simulink model "pitch_PD"  (R2013b)
settings: Solver=ode3  StartTime=0.0  StopTime=20  FixedStep=0.001  RelTol=1e-3
settings Model: Creator=Zhaolei  LastModifiedBy=Zhaolei

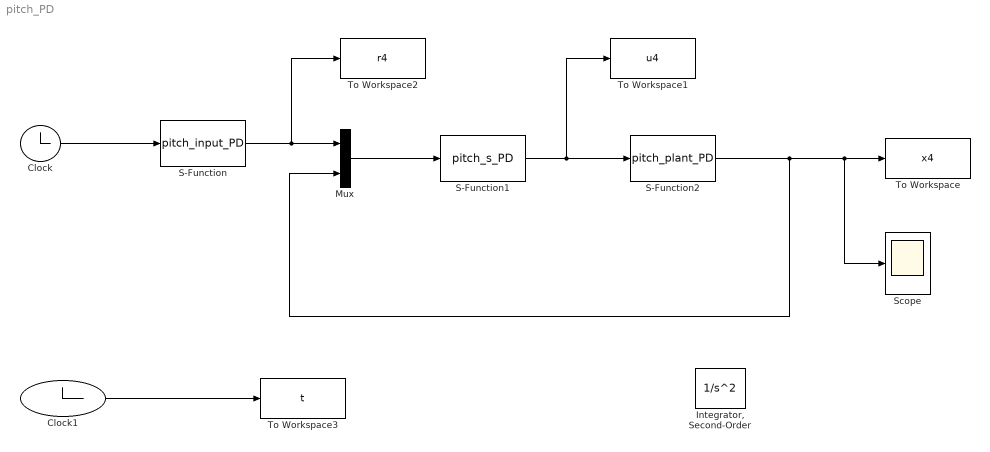
== system pitch_PD ==
  Clock : Clock
  Clock1 : Clock
  "Integrator, Second-Order" : SecondOrderIntegrator
  Mux : Mux  Inputs=2
  S-Function : S-Function  FunctionName=pitch_input_PD  EnableBusSupport=off
  S-Function1 : S-Function  FunctionName=pitch_s_PD  EnableBusSupport=off
  S-Function2 : S-Function  FunctionName=pitch_plant_PD  EnableBusSupport=off
  Scope : Scope
  To Workspace : ToWorkspace  VariableName=x4  SampleTime=-1
  To Workspace1 : ToWorkspace  VariableName=u4  SampleTime=-1
  To Workspace2 : ToWorkspace  VariableName=r4  SampleTime=-1
  To Workspace3 : ToWorkspace  VariableName=t  SampleTime=-1
  wires:
  Clock/1 -> S-Function/1
  Mux/1 -> S-Function1/1
  S-Function1/1 -> To Workspace1/1, S-Function2/1
  S-Function2/1 -> Mux/2, Scope/1, To Workspace/1
  Clock1/1 -> To Workspace3/1
  S-Function/1 -> To Workspace2/1, Mux/1
